simulink model "HW2"  (R2021a)
settings: Solver=VariableStepAuto  StartTime=0.0  StopTime=12  RelTol=1e-3
settings Model: Creator=thana  LastModifiedBy=thana

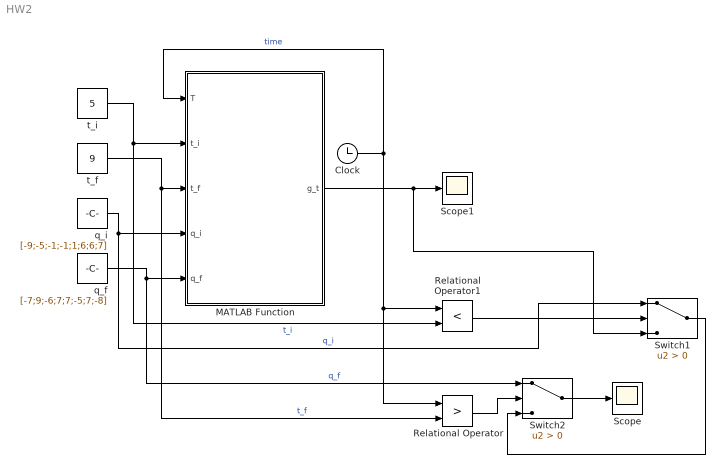
== system HW2 ==
  Clock : Clock
  MATLAB Function : MATLAB Function  TreatAsAtomicUnit=on
  Relational Operator : RelationalOperator  Operator=>  OutDataTypeStr=boolean  RndMeth=Simplest
  Relational Operator1 : RelationalOperator  Operator=<  OutDataTypeStr=boolean  RndMeth=Simplest
  Scope : Scope
  Scope1 : Scope
  Switch1 : Switch  Criteria=u2 > Threshold
  Switch2 : Switch  Criteria=u2 > Threshold
  q_f : Constant  Value=[-7;9;-6;7;7;-5;7;-8]  SampleTime=0
  q_i : Constant  Value=[-9;-5;-1;-1;1;6;6;7]
  t_f : Constant  Value=9  SampleTime=1
  t_i : Constant  Value=5  SampleTime=1
  wires:
  t_i/1 -> MATLAB Function/2(t_i), Relational Operator1/2  "t_i"
  t_f/1 -> Relational Operator/2, MATLAB Function/3(t_f)  "t_f"
  q_f/1 -> Switch2/1, MATLAB Function/5(q_f)  "q_f"
  q_i/1 -> MATLAB Function/4(q_i), Switch1/1  "q_i"
  Clock/1 -> MATLAB Function/1(T), Relational Operator/1, Relational Operator1/1  "time"
  Relational Operator/1 -> Switch2/2
  Relational Operator1/1 -> Switch1/2
  Switch1/1 -> Switch2/3
  Switch2/1 -> Scope/1
  MATLAB Function/1(g_t) -> Switch1/3, Scope1/1

== matlab function HW2/MATLAB Function ==
  data: T input; t_i input; g_t output; t_f input; q_i input; q_f input
function g_t = fcn(T,t_i,t_f,q_i,q_f)
c = zeros(numel(q_i),4);
%ax = axes;
%hold on ;
t1 = 0:0.01:t_i-0.01;
t2 = t_i:0.01:t_f;
t3 = t_f-0.01:0.01:t_f+t_i;
t = [t1 t2 t3]';
z = zeros(numel(t),numel(q_i));
for i = 1:numel(q_i)
    RHS = [q_i(i) ; q_f(i) ; 0 ; 0 ];
    A = [1 t_i (t_i^2) (t_i^3) ; 1 t_f (t_f^2) (t_f^3) ; 0 1 (2*t_i) (3*(t_i^2)) ;  0 1 (2*t_f) (3*(t_f^2))] ;
    ac0 = A ;
    ac0(:,1) = RHS';
    c_0 = det(ac0)/ det(A) ;
    ac1 = A ;
    ac1(:,2) = RHS';
    c_1 = det(ac1)/ det(A) ;
    ac2 = A ;
    ac2(:,3) = RHS';
    c_2 = det(ac2)/ det(A) ;
    ac3 = A ;
    ac3(:,4) = RHS';
    c_3 = det(ac3)/ det(A) ;
    c(i,:) = [c_3 c_2 c_1 c_0];
    %g_t = c_0 + c_1*T + c_2*(T.^2) + c_3*(T.^3) ;
    %{
    for j = 1:numel(t)
        if t(j) < t_i
            z(j,i) = q_i(i);
        elseif t(j) >= t_i && t(j) <= t_f
            z(j,i) = c_0 + c_1*t(j) + c_2*(t(j)^2) + c_3*(t(j)^3) ;
        else
            z(j,i) = q_f(i);
        end
    end
    %plot(ax,t,z(:,i));
    %}
    g_t = c(:,4) + c(:,3)*T + c(:,2)*(T.^2) + c(:,1)*(T.^3) ;
end
